simulink model "visualStateEstimator"  (R2024b)
settings: Solver=FixedStepAuto  StartTime=0.0  StopTime=10  FixedStep=0.1  RelTol=1e-3
InitFcn:
  | map = load(fullfile('.', '/Resources/map.mat'));
  | 
  | T_imu2rq = map.worldObjectStruct.transforms.T_imu2genquad;
  | R_imu2rq = T_imu2rq(1:3, 1:3);
  | t_imu2rq = T_imu2rq(1:3, 4);
  | 
  | T_rc2rq = map.worldObjectStruct.transforms.T_gencam2genquad;
  | R_rc2rq= T_rc2rq(1:3, 1:3);
  | t_rc2rq = T_rc2rq(1:3, 4);
  | 
  | T_uc2rc = map.worldObjectStruct.transforms.T_simcam2gencam;
  | R_uc2rc = T_uc2rc(1:3, 1:3);
  | 
  | T_uw2rw = map.worldObjectStruct.transforms.T_sim2world;
  | R_uw2rw = T_uw2rw(1:3, 1:3);
  | 
  | T_uq2rq = map.worldObjectStruct.transforms.T_simquad2genquad;
  | R_uq2rq = T_uq2rq(1:3, 1:3);
  | 
  | t_checker = map.worldObjectStruct.checkers(1).Position;
  | X_pnts_W = map.worldObjectStruct.checkers(1).Corners;
  | checkerSize = map.worldObjectStruct.checkers(1).NumSquares;
  | squareSize = map.worldObjectStruct.checkers(1).SquareSize;
  | 
  | 
  | simHz = simset.simHz;
  | imuHz = simset.imuHz;
  | imuHz = 1/(1/imuHz - rem((1/imuHz), (1/simHz)));
  | ekfHz = simset.ekfHz;
  | ekfHz = 1/(1/ekfHz - rem((1/ekfHz), (1/simHz)));
  | envHz = simset.envHz;
  | envHz = 1/(1/envHz - rem((1/envHz), (1/simHz)));
  | fps = simset.fps;
  | fps = 1/(1/fps - rem((1/fps), (1/envHz)));
  | if exist('imuWait', 'var') == 0
  |     imuWait = (1/simHz)*2;
  | end
  | 
  | K = camCalib_pin.K;
  | k_rad = camCalib_pin.radialDistortion;
  | k_tan = camCalib_pin.tangentialDistortion;
  | %p3pNode = ros2node('p3p_node', 2);
  | 
  | 
  | %pose_0 = [wp_pos_ts.Data(:,1,1); eul2quat(deg2rad(wp_eul_ts.Data(:,1,1))', 'XYZ')'];
  | pose_0 = [simset.pos0; eul2quat(simset.eul0', 'XYZ')'];
  | 
  | %setIMUParams;
StopFcn:
  | disp("Please save the flight log in QGroundControl")
settings Model: Creator=dylanfanner  LastModifiedBy=Alyssa
settings DataIOCC: SaveOutput=off  SaveTime=off
settings OptimizationCC: EnhancedBackFolding=on  PassReuseOutputArgsAs=Individual arguments  ZeroExternalMemoryAtStartup=off  ZeroInternalMemoryAtStartup=off  MaxStackSize=64  OptimizeBlockOrder=speed  DifferentSizesBufferReuse=on  OptimizationCustomize=off  EfficientTunableParamExpr=on
settings DebuggingCC: ParameterTunabilityLossMsg=error
settings HardwareCC: ProdBitPerLong=64  ProdHWDeviceType=Intel->x86-64 (Linux 64)
settings RTWCC: Description=Embedded Coder  SystemTargetFile=ert.tlc  HardwareBoard=Robot Operating System 2 (ROS 2)  TLCOptions="-aInlineSetEventsForThisBaseRateFcn=TLC_FALSE -aSuppressMultiTaskScheduler=TLC_FALSE  -aRateBasedStepFcn=0"  TemplateMakefile=ert_default_tmf  Toolchain=Colcon Tools  TargetLang=C++
settings CodeAppCC: ForceParamTrailComments=on  IgnoreCustomStorageClasses=off  OperatorAnnotations=on  SimulinkDataObjDesc=on  SFDataObjDesc=on  InsertBlockDesc=on
settings ERTTargetCC: CodeInterfacePackaging=C++ class  InlinedParameterPlacement=Hierarchical  RootIOFormat=Structure reference  DynamicArrayContainerType=coder::array

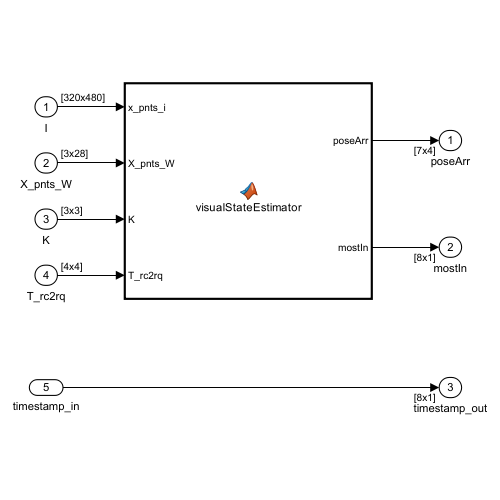
[thumbnail: Simulink's stored preview of the top-level diagram]
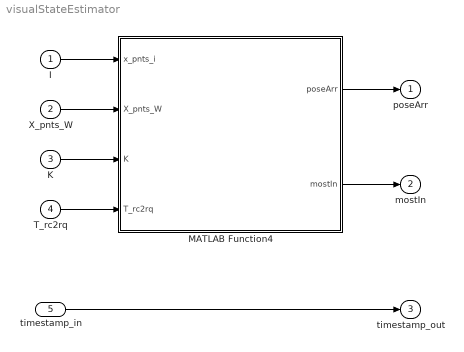
== system visualStateEstimator ==
  I : Inport  OutDataTypeStr=uint8  PortDimensions=[320 480]  SampleTime=[0.10000000000000001,0]
  X_pnts_W : Inport  Port=2  OutDataTypeStr=double  PortDimensions=[3 28]
  K : Inport  Port=3  OutDataTypeStr=double  PortDimensions=[3 3]
  T_rc2rq : Inport  Port=4  OutDataTypeStr=double  PortDimensions=[4 4]
  timestamp_in : Inport  Port=5
  MATLAB Function4 : MATLAB Function  TreatAsAtomicUnit=on
  poseArr : Outport  OutDataTypeStr=double  PortDimensions=[7 4]  SampleTime=[0.10000000000000001,0]
  mostIn : Outport  Port=2  OutDataTypeStr=double  PortDimensions=[8 1]  SampleTime=[0.10000000000000001,0]
  timestamp_out : Outport  Port=3  OutDataTypeStr=double  PortDimensions=[8 1]  SampleTime=[0.10000000000000001,0]
  wires:
  I/1 -> MATLAB Function4/1(x_pnts_i)
  X_pnts_W/1 -> MATLAB Function4/2(X_pnts_W)
  K/1 -> MATLAB Function4/3(K)
  T_rc2rq/1 -> MATLAB Function4/4(T_rc2rq)
  MATLAB Function4/1(poseArr) -> poseArr/1
  MATLAB Function4/2(mostIn) -> mostIn/1
  timestamp_in/1 -> timestamp_out/1

== matlab function visualStateEstimator/MATLAB Function4 ==
  data: x_pnts_i input uint8 size=[320,480]; poseArr output size=[7,4]; X_pnts_W input; K input; mostIn output size=[8,1]; T_rc2rq input
function [poseArr, mostIn] = visualStateEstimator(x_pnts_i, X_pnts_W, K, T_rc2rq)

%variables
inlierThreshold = 1;
poseArr = nan(7, 4);
mostIn = nan(8,1);
T_mostIn = nan(4,4);
soln = struct('T_arr', nan(4,4,4), 'poseArr', nan(7,4,4), 'mostInliers', struct('T', nan(4,4), 'Num', []), 'minReproj', struct('T', nan, 'Err', []));


%run Kneip's P3P
if ~isnan(x_pnts_i(1,1))
   
    soln = p3pRun.KneipN(x_pnts_i', X_pnts_W, K, checkerSize, inlierThreshold); %can be streamlined, currently much overhead: outputs struct with poses, Rt matrices, most inliers, least reproj...
    
    for j = 1:size(poseArr,2)
        poseArr(1:7,j) = soln.poseArr(1:7,j); %all rc2rw
        poseArr(1:3,j)= poseArr(1:3,j) * 1e-3; %convert to m
    end
    
    %some conversions
    T_mostIn(1:4, 1:4) = soln.mostInliers.T(1:4, 1:4); %position actually in mm
    T_mostIn(1:3, 4) = T_mostIn(1:3, 4) * 1e-3; %convert to m ; still rc2rw
    T_mostIn = T_mostIn * p3pFuncs.invertT(T_rc2rq);

    %and convert to pose
    mostIn(1:3,1) = T_mostIn(1:3, 4);
    mostIn(4:7,1) =tform2quat(T_mostIn)'; 
    mostIn(8,1) = soln.mostInliers.Num;
    %pose_minReproj =
end
